simulink model "dyn"  (R2022a)
settings: Solver=VariableStepAuto  StartTime=0.0  StopTime=10.0  RelTol=1e-3
settings Model: Creator=izacu  LastModifiedBy=izacu

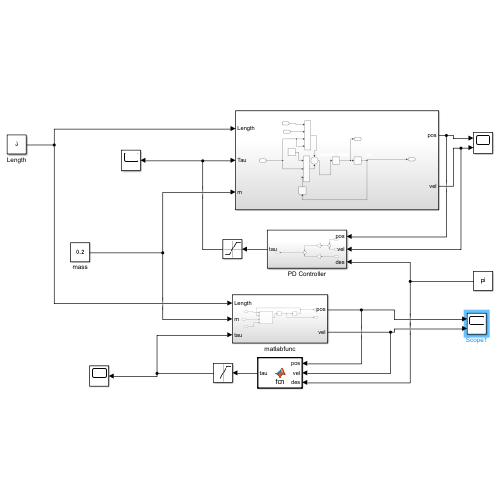
[thumbnail: Simulink's stored preview of the top-level diagram]
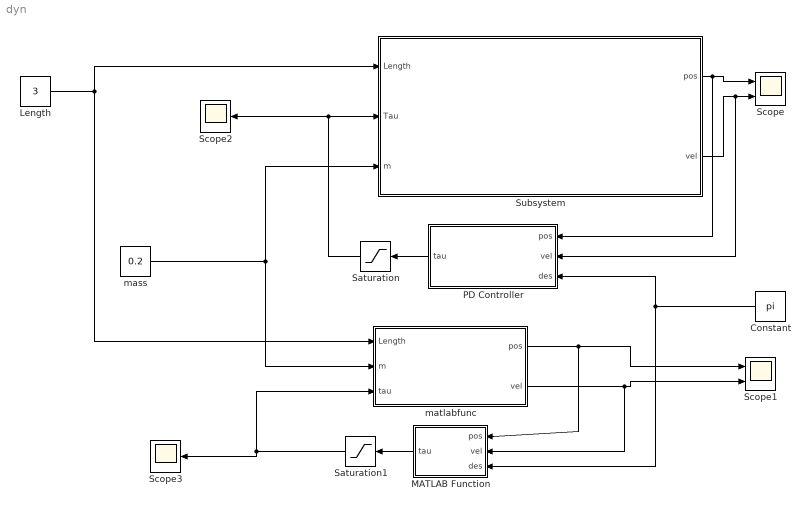
== system dyn ==
  Constant : Constant  Value=pi
  Length : Constant  Value=3
  MATLAB Function : MATLAB Function  TreatAsAtomicUnit=on
  PD Controller : Subsystem
  Saturation : Saturate  UpperLimit=8  LowerLimit=-8
  Saturation1 : Saturate  UpperLimit=8  LowerLimit=-8
  Scope : Scope  NumInputPorts=2
  Scope1 : Scope  NumInputPorts=2
  Scope2 : Scope
  Scope3 : Scope
  Subsystem : Subsystem
  mass : Constant  Value=0.2
  matlabfunc : Subsystem
  wires:
  matlabfunc/1(pos) -> Scope1/1, MATLAB Function/1(pos)
  matlabfunc/2(vel) -> MATLAB Function/2(vel), Scope1/2
  Length/1 -> matlabfunc/1(Length), Subsystem/1(Length)
  Subsystem/1(pos) -> Scope/1, PD Controller/1(pos)
  Subsystem/2(vel) -> PD Controller/2(vel), Scope/2
  mass/1 -> matlabfunc/2(m), Subsystem/3(m)
  PD Controller/1(tau) -> Saturation/1
  MATLAB Function/1(tau) -> Saturation1/1
  Constant/1 -> MATLAB Function/3(des), PD Controller/3(des)
  Saturation/1 -> Scope2/1, Subsystem/2(Tau)
  Saturation1/1 -> matlabfunc/3(tau), Scope3/1

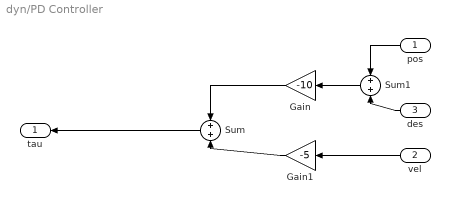
== system dyn/PD Controller ==
  pos : Inport
  vel : Inport  Port=2
  des : Inport  Port=3
  Gain : Gain  Gain=-10
  Gain1 : Gain  Gain=-5
  Sum : Sum
  Sum1 : Sum
  tau : Outport
  wires:
  Sum/1 -> tau/1
  vel/1 -> Gain1/1
  Gain/1 -> Sum/1
  Gain1/1 -> Sum/2
  Sum1/1 -> Gain/1
  des/1 -> Sum1/2
  pos/1 -> Sum1/1

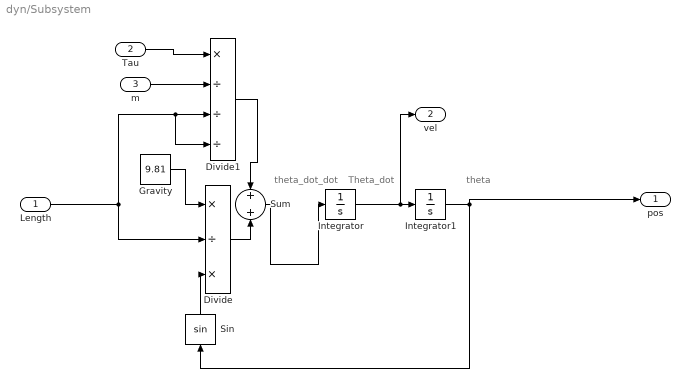
== system dyn/Subsystem ==
  note: theta
  note: Theta_dot
  note: theta_dot_dot
  Length : Inport
  Tau : Inport  Port=2
  m : Inport  Port=3
  Divide : Product  Inputs=*/*
  Divide1 : Product  Inputs=*///
  Gravity : Constant  Value=9.81
  Integrator : Integrator
  Integrator1 : Integrator  InitialCondition=pi/3
  Sin : Trigonometry
  Sum : Sum
  pos : Outport
  vel : Outport  Port=2
  wires:
  Gravity/1 -> Divide/1
  Integrator1/1 -> pos/1, Sin/1
  Integrator/1 -> vel/1, Integrator1/1
  Sin/1 -> Divide/3
  Length/1 -> Divide1/4, Divide1/3, Divide/2
  m/1 -> Divide1/2
  Tau/1 -> Divide1/1
  Divide/1 -> Sum/2
  Divide1/1 -> Sum/1
  Sum/1 -> Integrator/1

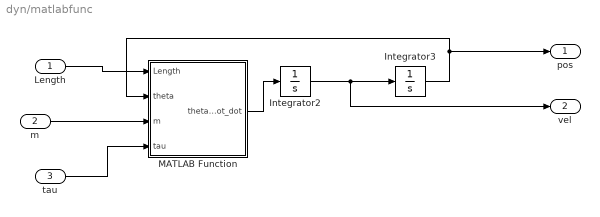
== system dyn/matlabfunc ==
  Length : Inport
  m : Inport  Port=2
  tau : Inport  Port=3
  Integrator2 : Integrator
  Integrator3 : Integrator  InitialCondition=pi/3
  MATLAB Function : MATLAB Function  TreatAsAtomicUnit=on
  pos : Outport
  vel : Outport  Port=2
  wires:
  Integrator2/1 -> vel/1, Integrator3/1
  MATLAB Function/1(theta_dot_dot) -> Integrator2/1
  Integrator3/1 -> pos/1, MATLAB Function/2(theta)
  Length/1 -> MATLAB Function/1(Length)
  m/1 -> MATLAB Function/3(m)
  tau/1 -> MATLAB Function/4(tau)

== matlab function dyn/MATLAB Function ==
  data: pos input; tau output; vel input; des input
function tau = fcn(pos,vel,des)

tau = -10 * (pos - des) - 5 * (vel - des);

== matlab function dyn/matlabfunc/MATLAB Function ==
  data: Length input; theta input; theta_dot_dot output; m input; tau input
function theta_dot_dot = dyn(Length, theta,m,tau)
g = 9.81;
len  = Length;

theta_dot_dot = -(g/len) * sin(theta) + tau/m/len^2;
